simulink model "dif_eq_in_simulin"  (R2024b)
settings: Solver=VariableStepAuto  StartTime=0.0  StopTime=10.0  RelTol=1e-3
settings Model: Creator=darkk157night  LastModifiedBy=darkk157night

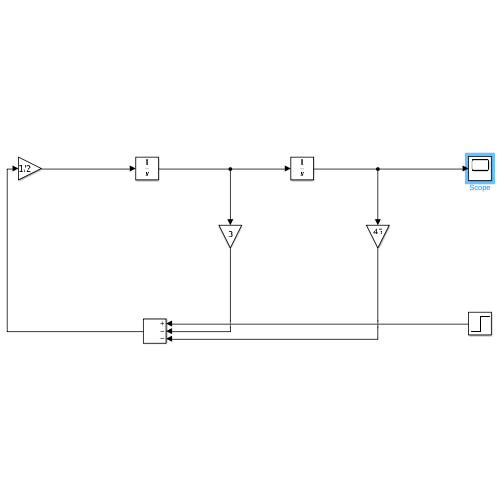
[thumbnail: Simulink's stored preview of the top-level diagram]
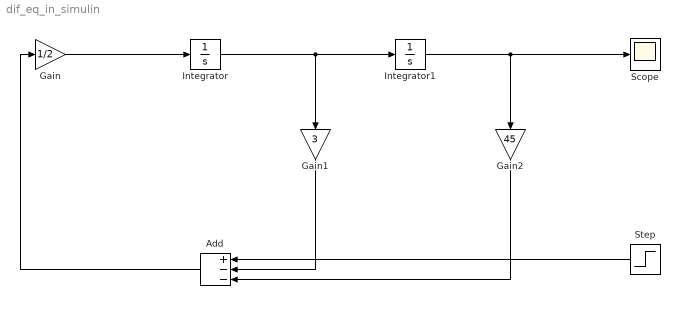
== system dif_eq_in_simulin ==
  Add : Sum  Inputs=+--
  Gain : Gain  Gain=1/2
  Gain1 : Gain  Gain=3
  Gain2 : Gain  Gain=45
  Integrator : Integrator
  Integrator1 : Integrator
  Scope : Scope
  Step : Step  After=90  SampleTime=0
  wires:
  Gain/1 -> Integrator/1
  Integrator/1 -> Integrator1/1, Gain1/1
  Integrator1/1 -> Gain2/1, Scope/1
  Gain2/1 -> Add/3
  Gain1/1 -> Add/2
  Step/1 -> Add/1
  Add/1 -> Gain/1
